simulink model "chap3_2sim"  (Simulink 7.7)
settings: Solver=ode45  SolverMode=SingleTasking  StartTime=0.0  StopTime=30  FixedStep=0.001  RelTol=1e-3
settings Model: Creator=ljk  LastModifiedBy=ljk  ExtModeTrigMode=oneshot  ExtModeArmWhenConnect=off
settings DataIOCC: LimitDataPoints=off  SignalLoggingName=sigsOut
settings OptimizationCC: BooleanDataType=off
settings DebuggingCC: SaveWithParameterizedLinksMsg=none  SignalResolutionControl=TryResolveAllWithWarning  SolverPrmCheckMsg=none  MultiTaskDSMMsg=warning  MultiTaskCondExecSysMsg=none  StrictBusMsg=None
settings HardwareCC: TargetUnknown=on
settings RTWCC: IncludeERTFirstTime=on

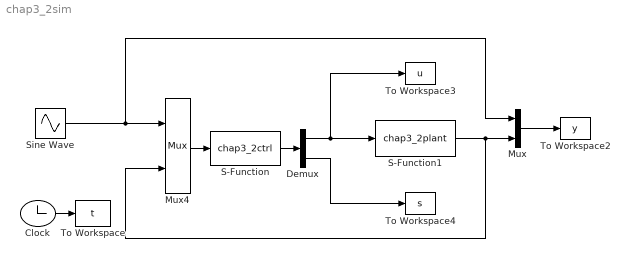
== system chap3_2sim ==
  Clock : Clock
  Demux : Demux  Outputs=2
  Mux : Mux  Inputs=2
  Mux4 : Mux  Inputs=2
  S-Function : S-Function  FunctionName=chap3_2ctrl  EnableBusSupport=off
  S-Function1 : S-Function  FunctionName=chap3_2plant  EnableBusSupport=off
  Sine Wave : Sin  SampleTime=0
  To Workspace : ToWorkspace  VariableName=t  SampleTime=-1  SaveFormat=Array
  To Workspace2 : ToWorkspace  VariableName=y  SampleTime=-1  SaveFormat=Array
  To Workspace3 : ToWorkspace  VariableName=u  SampleTime=-1  SaveFormat=Array
  To Workspace4 : ToWorkspace  VariableName=s  SampleTime=-1  SaveFormat=Array
  wires:
  Mux4/1 -> S-Function/1
  Clock/1 -> To Workspace/1
  Sine Wave/1 -> Mux/1, Mux4/1
  S-Function/1 -> Demux/1
  S-Function1/1 -> Mux4/2, Mux/2
  Mux/1 -> To Workspace2/1
  Demux/1 -> S-Function1/1, To Workspace3/1
  Demux/2 -> To Workspace4/1
